simulink model "bh_SM_quad_NO_spin_props"  (R2017a)
settings: Solver=ode23t  StartTime=0.0  StopTime=200  FixedStep=0.001  RelTol=1e-5  EnableMultiTasking=on
undefined symbols (not defined in the file): P_elec, P_mot, P_one_prop, P_rot, P_veh, P_veh_no_props, sigbuilder_block, X, xme_dot_0, Y, Z
libraries: bh_6dof_LIBRARY x22, sm_lib x22, nesl_utility x19, simulink_extras x17, simulink x15
(part 3 of 3)

== system bh_SM_quad_NO_spin_props/CONT_SYS W_MOT_CMDS/MOTOR_sys/MOTOR_1/prefilter ==
  note: Y = U *     wn^2/( s^2 + 2*p*wn*s + wn^2)
      | Y*( s^2 + 2*p*wn*s + wn^2) = U * wn^2
      |
      | y'' + y'*2*p*wn + y*wn^2 = U*wn^2
  U : Inport
  Gain : Gain  Gain=2*p*wn
  Gain1 : Gain  Gain=wn^2
  Gain2 : Gain  Gain=wn^2
  Integrator : Integrator
  Integrator1 : Integrator
  Sum : Sum  Inputs=|+--
  U_filt : Outport
  U_DOT : Outport  Port=2
  wires:
  Integrator/1 -> Integrator1/1, [Y_DOT], Gain/1  "y_dot"
  Sum/1 -> Integrator/1  "y_dot_dot"
  Integrator1/1 -> Gain1/1, U_filt/1  "y"
  U/1 -> Gain2/1
  Gain2/1 -> Sum/1
  Gain/1 -> Sum/3
  Gain1/1 -> Sum/2
  [Y_DOT] -> U_DOT/1

== system bh_SM_quad_NO_spin_props/CONT_SYS W_MOT_CMDS/MOTOR_sys/MOTOR_2/prefilter ==
  note: Y = U *     wn^2/( s^2 + 2*p*wn*s + wn^2)
      | Y*( s^2 + 2*p*wn*s + wn^2) = U * wn^2
      |
      | y'' + y'*2*p*wn + y*wn^2 = U*wn^2
  U : Inport
  Gain : Gain  Gain=2*p*wn
  Gain1 : Gain  Gain=wn^2
  Gain2 : Gain  Gain=wn^2
  Integrator : Integrator
  Integrator1 : Integrator
  Sum : Sum  Inputs=|+--
  U_filt : Outport
  U_DOT : Outport  Port=2
  wires:
  Integrator/1 -> Integrator1/1, [Y_DOT], Gain/1  "y_dot"
  Sum/1 -> Integrator/1  "y_dot_dot"
  Integrator1/1 -> Gain1/1, U_filt/1  "y"
  U/1 -> Gain2/1
  Gain2/1 -> Sum/1
  Gain/1 -> Sum/3
  Gain1/1 -> Sum/2
  [Y_DOT] -> U_DOT/1

== system bh_SM_quad_NO_spin_props/CONT_SYS W_MOT_CMDS/MOTOR_sys/MOTOR_3/prefilter ==
  note: Y = U *     wn^2/( s^2 + 2*p*wn*s + wn^2)
      | Y*( s^2 + 2*p*wn*s + wn^2) = U * wn^2
      |
      | y'' + y'*2*p*wn + y*wn^2 = U*wn^2
  U : Inport
  Gain : Gain  Gain=2*p*wn
  Gain1 : Gain  Gain=wn^2
  Gain2 : Gain  Gain=wn^2
  Integrator : Integrator
  Integrator1 : Integrator
  Sum : Sum  Inputs=|+--
  U_filt : Outport
  U_DOT : Outport  Port=2
  wires:
  Integrator/1 -> Integrator1/1, [Y_DOT], Gain/1  "y_dot"
  Sum/1 -> Integrator/1  "y_dot_dot"
  Integrator1/1 -> Gain1/1, U_filt/1  "y"
  U/1 -> Gain2/1
  Gain2/1 -> Sum/1
  Gain/1 -> Sum/3
  Gain1/1 -> Sum/2
  [Y_DOT] -> U_DOT/1

== system bh_SM_quad_NO_spin_props/CONT_SYS W_MOT_CMDS/MOTOR_sys/MOTOR_4/prefilter ==
  note: Y = U *     wn^2/( s^2 + 2*p*wn*s + wn^2)
      | Y*( s^2 + 2*p*wn*s + wn^2) = U * wn^2
      |
      | y'' + y'*2*p*wn + y*wn^2 = U*wn^2
  U : Inport
  Gain : Gain  Gain=2*p*wn
  Gain1 : Gain  Gain=wn^2
  Gain2 : Gain  Gain=wn^2
  Integrator : Integrator
  Integrator1 : Integrator
  Sum : Sum  Inputs=|+--
  U_filt : Outport
  U_DOT : Outport  Port=2
  wires:
  Integrator/1 -> Integrator1/1, [Y_DOT], Gain/1  "y_dot"
  Sum/1 -> Integrator/1  "y_dot_dot"
  Integrator1/1 -> Gain1/1, U_filt/1  "y"
  U/1 -> Gain2/1
  Gain2/1 -> Sum/1
  Gain/1 -> Sum/3
  Gain1/1 -> Sum/2
  [Y_DOT] -> U_DOT/1

== system bh_SM_quad_NO_spin_props/MODEL_SYS/bh_6DOF (Simscape)/6DOF_JOINT_SYS/Angular_MEAS ==
  note: NOTE:  For the Transform sensor  block
      | Tthe DCM is:   r_BASE = R * r_FOLLOWER
  note: NOTE:  For the Transform sensor  block
      | The angular velocities are resolved into FOLLOWER frame components
  Calc Euler_rates : Subsystem
  Gain : Gain
  Math Function : Math  Operator=transpose  SaturateOnIntegerOverflow=on
  Mux : Mux  Inputs=3
  PS-Simulink Converter1 : nesl_utility/PS-Simulink Converter  PhysicalDomain=network_engine_domain  SubClassName=ps_output  LeftPortType=input  RightPortType=output  PseudoPeriodic=off  Frequencies=[]  Unit=rad/s  AffineConversion=off
  PS-Simulink Converter2 : nesl_utility/PS-Simulink Converter  PhysicalDomain=network_engine_domain  SubClassName=ps_output  LeftPortType=input  RightPortType=output  PseudoPeriodic=off  Frequencies=[]  Unit=rad/s  AffineConversion=off
  PS-Simulink Converter6 : nesl_utility/PS-Simulink Converter  PhysicalDomain=network_engine_domain  SubClassName=ps_output  LeftPortType=input  RightPortType=output  PseudoPeriodic=off  Frequencies=[]  Unit=1  AffineConversion=off
  PS-Simulink Converter7 : nesl_utility/PS-Simulink Converter  PhysicalDomain=network_engine_domain  SubClassName=ps_output  LeftPortType=input  RightPortType=output  PseudoPeriodic=off  Frequencies=[]  Unit=rad/s  AffineConversion=off
  Reshape1 : Reshape  OutputDimensionality=Column vector (2-D)
  Reshape2 : Reshape  OutputDimensionality=Column vector (2-D)
  Reshape3 : Reshape  OutputDimensionality=Column vector (2-D)
  Transform Sensor : sm_lib/Frames and Transforms/Transform Sensor  MeasurementFrame=Base  SenseAngle=off  SenseAxis=off  SenseAngle1=off  SenseAngle2=off  SenseAngle3=off  SenseQ=off  SenseR=on  SenseOmegaX=off  SenseOmegaY=off  SenseOmegaZ=off  SenseOmega1=off  SenseOmega2=off  SenseOmega3=off  SenseQDot=off  SenseRDot=off  SenseAlphaX=off  SenseAlphaY=off  SenseAlphaZ=off  SenseAlpha1=off  SenseAlpha2=off  SenseAlpha3=off  SenseQDDot=off  SenseRDDot=off  SenseX=off  SenseY=off  SenseZ=off  SenseRad=off  SenseAzim=off  SenseDist=off  SenseInc=off  SenseXDot=off  SenseYDot=off  SenseZDot=off  SenseRadDot=off  SenseAzimDot=off  SenseDistDot=off  SenseIncDot=off  SenseXDDot=off  SenseYDDot=off  SenseZDDot=off  SenseRadDDot=off  SenseAzimDDot=off  SenseDistDDot=off  SenseIncDDot=off
  Transform Sensor1 : sm_lib/Frames and Transforms/Transform Sensor  MeasurementFrame=Follower  SenseAngle=off  SenseAxis=off  SenseAngle1=off  SenseAngle2=off  SenseAngle3=off  SenseQ=off  SenseR=off  SenseOmegaX=on  SenseOmegaY=on  SenseOmegaZ=on  SenseOmega1=off  SenseOmega2=off  SenseOmega3=off  SenseQDot=off  SenseRDot=off  SenseAlphaX=off  SenseAlphaY=off  SenseAlphaZ=off  SenseAlpha1=off  SenseAlpha2=off  SenseAlpha3=off  SenseQDDot=off  SenseRDDot=off  SenseX=off  SenseY=off  SenseZ=off  SenseRad=off  SenseAzim=off  SenseDist=off  SenseInc=off  SenseXDot=off  SenseYDot=off  SenseZDot=off  SenseRadDot=off  SenseAzimDot=off  SenseDistDot=off  SenseIncDot=off  SenseXDDot=off  SenseYDDot=off  SenseZDDot=off  SenseRadDDot=off  SenseAzimDDot=off  SenseDistDDot=off  SenseIncDDot=off
  calc_DCM : MATLAB Function  TreatAsAtomicUnit=on
  B : PMIOPort  Port=1  Side=Left
  F : PMIOPort  Port=2  Side=Right
  wb : Outport
  bRg : Outport  Port=2
  eul : Outport  Port=3
  eul_rates : Outport  Port=4
  wires:
  PS-Simulink Converter6/1 -> Gain/1  "BRF"
  PS-Simulink Converter7/1 -> Mux/1
  PS-Simulink Converter1/1 -> Mux/2
  PS-Simulink Converter2/1 -> Mux/3
  Gain/1 -> Math Function/1  "gRb"
  Math Function/1 -> [bRg], bRg/1  "bRg"
  Mux/1 -> Reshape1/1
  [bRg] -> calc_DCM/1(bRg)
  calc_DCM/1(eul_vec) -> Reshape2/1
  Reshape2/1 -> [e], eul/1
  Calc Euler_rates/1(Euler_rates) -> Reshape3/1
  Reshape3/1 -> eul_rates/1
  Reshape1/1 -> [wb], wb/1
  [wb] -> Calc Euler_rates/1("p q r ")
  [e] -> Calc Euler_rates/2(Euler_angs)
  connections:
  PS-Simulink Converter7/LConn1 -- Transform Sensor1/RConn2
  PS-Simulink Converter6/LConn1 -- Transform Sensor/RConn2
  Transform Sensor1/RConn1 -- Transform Sensor/RConn1 -- F/RConn1
  Transform Sensor/LConn1 -- B/RConn1 -- Transform Sensor1/LConn1
  PS-Simulink Converter2/LConn1 -- Transform Sensor1/RConn4
  Transform Sensor1/RConn3 -- PS-Simulink Converter1/LConn1

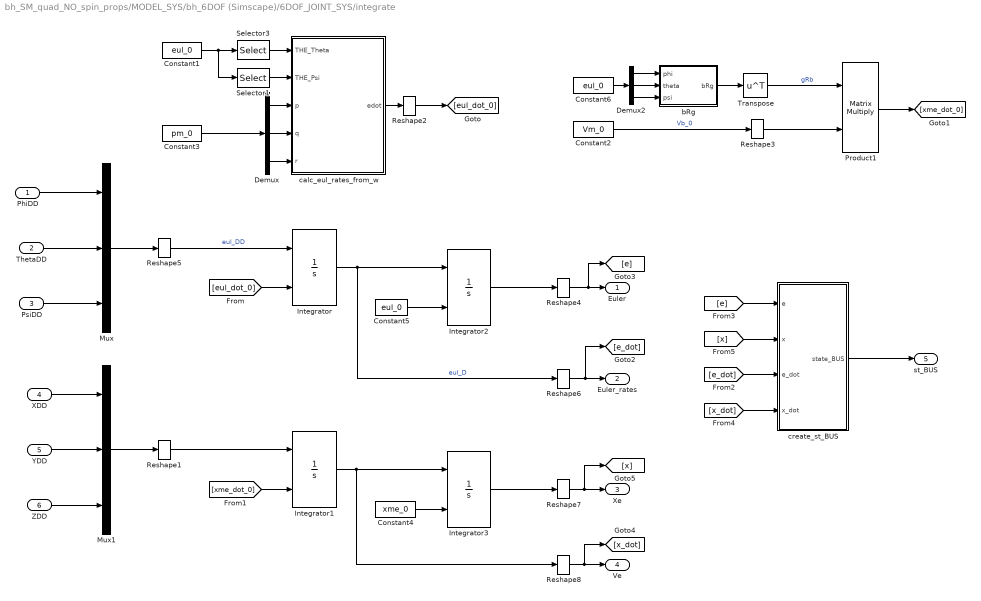
== system bh_SM_quad_NO_spin_props/MODEL_SYS/bh_6DOF (Simscape)/6DOF_JOINT_SYS/integrate ==
  PhiDD : Inport
  ThetaDD : Inport  Port=2
  PsiDD : Inport  Port=3
  XDD : Inport  Port=4
  YDD : Inport  Port=5
  ZDD : Inport  Port=6
  Constant1 : Constant  Value=eul_0  OutDataTypeStr=Inherit: Inherit via back propagation
  Constant2 : Constant  Value=Vm_0  OutDataTypeStr=Inherit: Inherit via back propagation
  Constant3 : Constant  Value=pm_0  OutDataTypeStr=Inherit: Inherit via back propagation
  Constant4 : Constant  Value=xme_0  OutDataTypeStr=Inherit: Inherit via back propagation
  Constant5 : Constant  Value=eul_0  OutDataTypeStr=Inherit: Inherit via back propagation
  Constant6 : Constant  Value=eul_0  OutDataTypeStr=Inherit: Inherit via back propagation
  Demux : Demux  Outputs=3
  Demux2 : Demux  Outputs=3
  Integrator : Integrator  InitialConditionSource=external  ContinuousStateAttributes={'DOT_phi', 'DOT_theta','DOT_psi'}
      settings: AttributesFormatString=%<ContinuousStateAttributes>
  Integrator1 : Integrator  InitialConditionSource=external  ContinuousStateAttributes={'DOT_Xe', 'DOT_Ye', 'DOT_Ze'}
      settings: AttributesFormatString=%<ContinuousStateAttributes>
  Integrator2 : Integrator  InitialConditionSource=external  ContinuousStateAttributes={'phi', 'theta','psi'}
      settings: AttributesFormatString=%<ContinuousStateAttributes>
  Integrator3 : Integrator  InitialConditionSource=external  ContinuousStateAttributes={'Xe', 'Ye', 'Ze'}
      settings: AttributesFormatString=%<ContinuousStateAttributes>
  Mux : Mux  Inputs=3
  Mux1 : Mux  Inputs=3
  Product1 : Product  Multiplication=Matrix(*)  SaturateOnIntegerOverflow=on  InputSameDT=on  OutDataTypeStr=Inherit: Same as first input
  Reshape{1..8} (8 alike) : Reshape  OutputDimensionality=Column vector (2-D)
  Selector1 : Selector  InputPortWidth=3  IndexOptions=Index vector (dialog)  Indices=3  OutputSizes=1
  Selector3 : Selector  InputPortWidth=3  IndexOptions=Index vector (dialog)  Indices=2  OutputSizes=1
  Transpose : Math  Operator=transpose  SaturateOnIntegerOverflow=on
  bRg : MATLAB Function  TreatAsAtomicUnit=on
  calc_eul_rates_from_w : MATLAB Function  TreatAsAtomicUnit=on
  create_st_BUS : Subsystem
  Euler : Outport
  Euler_rates : Outport  Port=2
  Xe : Outport  Port=3
  Ve : Outport  Port=4
  st_BUS : Outport  Port=5
  wires:
  PhiDD/1 -> Mux/1
  ThetaDD/1 -> Mux/2
  PsiDD/1 -> Mux/3
  Mux/1 -> Reshape5/1
  XDD/1 -> Mux1/1
  YDD/1 -> Mux1/2
  ZDD/1 -> Mux1/3
  Mux1/1 -> Reshape1/1
  Integrator1/1 -> Reshape8/1, Integrator3/1
  Integrator/1 -> Reshape6/1, Integrator2/1  "eul_D"
  Reshape5/1 -> Integrator/1  "eul_DD"
  Reshape1/1 -> Integrator1/1
  Constant5/1 -> Integrator2/2
  Constant1/1 -> Selector1/1, Selector3/1
  [eul_dot_0] -> Integrator/2
  Constant4/1 -> Integrator3/2
  Constant2/1 -> Reshape3/1  "Vb_0"
  bRg/1(bRg) -> Transpose/1
  Reshape3/1 -> Product1/2
  Constant6/1 -> Demux2/1
  Transpose/1 -> Product1/1  "gRb"
  Product1/1 -> [xme_dot_0]
  [xme_dot_0] -> Integrator1/2
  Integrator3/1 -> Reshape7/1
  Integrator2/1 -> Reshape4/1
  Reshape4/1 -> [e], Euler/1
  Reshape6/1 -> [e_dot], Euler_rates/1
  Reshape7/1 -> [x], Xe/1
  Reshape8/1 -> [x_dot], Ve/1
  Demux2/1 -> bRg/1(phi)
  Demux2/2 -> bRg/2(theta)
  Demux2/3 -> bRg/3(psi)
  Selector3/1 -> calc_eul_rates_from_w/1(THE_Theta)
  Selector1/1 -> calc_eul_rates_from_w/2(THE_Psi)
  Demux/3 -> calc_eul_rates_from_w/5(r)
  Demux/2 -> calc_eul_rates_from_w/4(q)
  Demux/1 -> calc_eul_rates_from_w/3(p)
  calc_eul_rates_from_w/1(edot) -> Reshape2/1
  Constant3/1 -> Demux/1
  Reshape2/1 -> [eul_dot_0]
  [e] -> create_st_BUS/1(e)
  [x] -> create_st_BUS/2(x)
  [e_dot] -> create_st_BUS/3(e_dot)
  [x_dot] -> create_st_BUS/4(x_dot)
  create_st_BUS/1(state_BUS) -> st_BUS/1

== system bh_SM_quad_NO_spin_props/MODEL_SYS/bh_6DOF (Simscape)/6DOF_JOINT_SYS/Angular_MEAS/Calc Euler_rates ==
  "p q r " : Inport
  Euler_angs : Inport  Port=2
  Demux1 : Demux  Outputs=3
  Demux2 : Demux  Outputs=3
  Demux3 : Demux  Outputs=3
  Mux1 : Mux  Inputs=3
  Reshape1 : Reshape  OutputDimensionality=Column vector (2-D)
  Reshape2 : Reshape  OutputDimensionality=Column vector (2-D)
  Terminator : Terminator
  my_euler_rates : MATLAB Function  TreatAsAtomicUnit=on
  Euler_rates : Outport
  wires:
  Reshape1/1 -> Demux3/1  "wb"
  my_euler_rates/1(euler_rates) -> Demux2/1  "euler_rates"
  Demux2/3 -> Mux1/3  "psidot_X3_roll"
  Demux2/2 -> Mux1/2  "thetadot_Y2_pitch"
  Demux2/1 -> Mux1/1  "phidot_Z1_yaw"
  Reshape2/1 -> Euler_rates/1
  Mux1/1 -> Reshape2/1
  Demux3/3 -> my_euler_rates/5(r)
  Demux3/2 -> my_euler_rates/4(q)
  Demux3/1 -> my_euler_rates/3(p)
  Euler_angs/1 -> Demux1/1
  "p q r "/1 -> Reshape1/1
  Demux1/2 -> my_euler_rates/1(theta)  "theta"
  Demux1/1 -> Terminator/1  "phi"
  Demux1/3 -> my_euler_rates/2(psi)  "psi"

== system bh_SM_quad_NO_spin_props/MODEL_SYS/bh_6DOF (Simscape)/6DOF_JOINT_SYS/integrate/create_st_BUS ==
  e : Inport
  x : Inport  Port=2
  e_dot : Inport  Port=3
  x_dot : Inport  Port=4
  Bus Creator : BusCreator  Inputs=4
  Bus Creator1 : BusCreator  Inputs=6
  Bus Creator2 : BusCreator  Inputs=6
  Demux{,1..3} (4 alike) : Demux  Outputs=3
  Mux : Mux  Inputs=2
  Mux1 : Mux  Inputs=2
  Reshape1 : Reshape  OutputDimensionality=Column vector (2-D)
  Reshape8 : Reshape  OutputDimensionality=Column vector (2-D)
  state_BUS : Outport
  wires:
  e/1 -> Mux/1, [e]
  x/1 -> Mux/2, [x]
  e_dot/1 -> Mux1/1, [eD]
  x_dot/1 -> Mux1/2, [xD]
  Mux1/1 -> Reshape1/1
  Mux/1 -> Reshape8/1
  Reshape1/1 -> Bus Creator/2  "vel_col"
  Reshape8/1 -> Bus Creator/1  "pos_col"
  Bus Creator1/1 -> Bus Creator/3  "Pos_list"
  Demux/1 -> Bus Creator1/1  "Phi"
  Demux/2 -> Bus Creator1/2  "Theta"
  Demux/3 -> Bus Creator1/3  "Psi"
  Demux1/2 -> Bus Creator1/5  "Y"
  Demux1/3 -> Bus Creator1/6  "Z"
  Demux1/1 -> Bus Creator1/4  "X"
  [e] -> Demux/1
  [x] -> Demux1/1
  Bus Creator2/1 -> Bus Creator/4  "Vel_list"
  Demux2/1 -> Bus Creator2/1  "Phi_D"
  Demux2/2 -> Bus Creator2/2  "Theta_D"
  Demux2/3 -> Bus Creator2/3  "Psi_D"
  Demux3/1 -> Bus Creator2/4  "X_D"
  Demux3/2 -> Bus Creator2/5  "Y_D"
  Demux3/3 -> Bus Creator2/6  "Z_D"
  [eD] -> Demux2/1
  [xD] -> Demux3/1
  Bus Creator/1 -> state_BUS/1

== matlab function bh_SM_quad_NO_spin_props/MODEL_SYS/bh_6DOF (Simscape)/6DOF_JOINT_SYS/integrate/bRg ==
  data: phi input; bRg output; theta input; psi input
function bRg = bRg(phi,theta,psi)
%#codegen

%    This function was generated by the Symbolic Math Toolbox version 7.2.
%    28-Aug-2017 10:05:16

bRg = reshape([cos(phi).*cos(theta),-cos(psi).*sin(phi)+cos(phi).*sin(psi).*sin(theta),sin(phi).*sin(psi)+cos(phi).*cos(psi).*sin(theta),cos(theta).*sin(phi),cos(phi).*cos(psi)+sin(phi).*sin(psi).*sin(theta),-cos(phi).*sin(psi)+cos(psi).*sin(phi).*sin(theta),-sin(theta),cos(theta).*sin(psi),cos(psi).*cos(theta)],[3,3]);

== matlab function bh_SM_quad_NO_spin_props/CONT_SYS W_MOT_CMDS/FM_to_w2 ==
  data: L input; w2_cmd output; Thrust_const input; Twist_const input; Thrust input; TQ_roll_X input; TQ_pit_Y input; TQ_yaw_Z input
function w2_cmd = FMtow2(L, Thrust_const, Twist_const, Thrust, TQ_roll_X, TQ_pit_Y, TQ_yaw_Z)
%#codegen

    % simplify the variable names
    b = Thrust_const;
    k = Twist_const;

    % construct the co-efficient matrix:
    %  F_and_M = C * w^2
    %
    % C = [     b,    b,    b,    b;
    %           0,    b*L,  0,   -b*L;
    %          -b*L,  0,    b*L,  0;
    %          -k,    k,   -k,    k; ];

    % used Symbolic toolbox to compute inv(C)
    C_inv = [
             1/(4*b),          0, -1/(2*L*b), -1/(4*k);
             1/(4*b),  1/(2*L*b),          0,  1/(4*k);
             1/(4*b),          0,  1/(2*L*b), -1/(4*k);
             1/(4*b), -1/(2*L*b),          0,  1/(4*k);
            ];
    % solve for the w^2 vec
    F_and_M_col = [Thrust, TQ_roll_X, TQ_pit_Y, TQ_yaw_Z].' ;

    w2_cmd = C_inv * F_and_M_col;
    
    tf_col = (w2_cmd >= 0);
   assert(all(w2_cmd), 'ERROR: some w2 are NEGATIVE !')
   %assert(false, 'ERROR: some w2 are NEGATIVE !')
end

== matlab function bh_SM_quad_NO_spin_props/a_circle1/MATLAB Function ==
  data: t_clock input; XYZ output; t_to_start input; RADIUS input; ztgt input; w input
function XYZ = fcn(t_clock, t_to_start, RADIUS, ztgt, w)

t    = t_clock - t_to_start;

theta = w*t;

x = RADIUS * cos(theta);
y = RADIUS * sin(theta);
z = ztgt;


XYZ = [x;y;z];

== matlab function bh_SM_quad_NO_spin_props/CONT_SYS Force_Moment_CMDS/PITCH_and_ROLL_CONT/MATLAB Function ==
  data: Gr input size=[2 1]; Qr output size=[2 1]; ang input size=[1 1]
function Qr = fcn(Gr, ang)
%#codegen

    bRg = [  cos(ang),  sin(ang);
            -sin(ang),  cos(ang);
          ];  

    Qr = bRg * Gr;
end

== matlab function bh_SM_quad_NO_spin_props/MODEL_SYS/bh_6DOF (Simscape)/6DOF_JOINT_SYS/Angular_MEAS/Calc Euler_rates/my_euler_rates ==
  data: theta input; euler_rates output; psi input; p input; q input; r input
function euler_rates = my_euler_rates(theta,psi,p,q,r)
%#codegen

%    This function was generated by the Symbolic Math Toolbox version 7.0.
%    09-Jun-2016 10:28:25

euler_rates = [(r.*cos(psi)+q.*sin(psi))./cos(theta);
                q.*cos(psi)-r.*sin(psi);
               (p.*cos(theta)+r.*cos(psi).*sin(theta)+q.*sin(psi).*sin(theta))./cos(theta)];

== matlab function bh_SM_quad_NO_spin_props/MODEL_SYS/bh_6DOF (Simscape)/6DOF_JOINT_SYS/integrate/calc_eul_rates_from_w ==
  data: THE_Theta input; edot output; THE_Psi input; p input; q input; r input
function edot = calc_eul_rates_from_w(THE_Theta,THE_Psi,p,q,r)
%#codegen

%    This function was generated by the Symbolic Math Toolbox version 7.2.
%    28-Aug-2017 10:05:22

edot = [(r.*cos(THE_Psi)+q.*sin(THE_Psi))./cos(THE_Theta);q.*cos(THE_Psi)-r.*sin(THE_Psi);(p.*cos(THE_Theta)+r.*cos(THE_Psi).*sin(THE_Theta)+q.*sin(THE_Psi).*sin(THE_Theta))./cos(THE_Theta)];

== matlab function bh_SM_quad_NO_spin_props/MODEL_SYS/bh_6DOF (Simscape)/6DOF_JOINT_SYS/Angular_MEAS/calc_DCM ==
  data: bRg input; eul_vec output
function eul_vec = calc_eul_ang(bRg)
%#codegen

% bRg = [ ...
%                               cos(phi)*cos(theta),                              cos(theta)*sin(phi),         -sin(theta);
%  cos(phi)*sin(psi)*sin(theta) - cos(psi)*sin(phi), cos(phi)*cos(psi) + sin(phi)*sin(psi)*sin(theta), cos(theta)*sin(psi);
%  sin(phi)*sin(psi) + cos(phi)*cos(psi)*sin(theta), cos(psi)*sin(phi)*sin(theta) - cos(phi)*sin(psi), cos(psi)*cos(theta);
%  ];

%phi, theta, psi


theta = asin( -bRg(1,3)  ); %  theta is in the range [-pi/2, pi/2]

% Recall the DOC on atan2()
%     atan2(Y,X) is the four quadrant arctangent of the elements of X and Y
%     such that -pi <= atan2(Y,X) <= pi

Y   = bRg(1,2);
X   = bRg(1,1);
phi = atan2(Y,X);

Y   = bRg(2,3);
X   = bRg(3,3);
psi = atan2(Y,X);

% now populate the output
eul_vec    = zeros(3,1);

eul_vec(1) = phi;
eul_vec(2) = theta;
eul_vec(3) = psi;

end

== matlab function bh_SM_quad_NO_spin_props/CONT_SYS W_MOT_CMDS/w2toFM1 ==
  data: L input; Tbz_col output; Thrust_const input; Twist_const input; w2_col input; Mbz_col output; wM_col output
function [Tbz_col, Mbz_col, wM_col] = w2toFM(L, Thrust_const, Twist_const, w2_col)
%#codegen

    % simplify the variable names
    b = Thrust_const;
    k = Twist_const;

    % construct the co-efficient matrix:
    %  F_and_M = C * w^2
    
%     C = [     b,    b,    b,    b;
%               0,    b*L,  0,   -b*L;
%              -b*L,  0,    b*L,  0;
%              -k,    k,   -k,    k; ];

    Tbz_col = [ b; b; b; b ]  .*  w2_col;     
    Mbz_col = [-k; k;-k; k ]  .*  w2_col;          
    wM_col  = [ 1;-1; 1;-1 ]  .*  sqrt(w2_col); 
end

== matlab function bh_SM_quad_NO_spin_props/CONT_SYS W_MOT_CMDS/w2toFM2 ==
  data: L input; Thrust output; Thrust_const input; Twist_const input; w2_col input; TQ_roll_X output; TQ_pit_Y output; TQ_yaw_Z output
function [Thrust, TQ_roll_X, TQ_pit_Y, TQ_yaw_Z] = w2toFM(L, Thrust_const, Twist_const, w2_col)
%#codegen

    % simplify the variable names
    b = Thrust_const;
    k = Twist_const;

    % construct the co-efficient matrix:
    %  F_and_M = C * w^2
    
    C = [     b,    b,    b,    b;
              0,    b*L,  0,   -b*L;
             -b*L,  0,    b*L,  0;
             -k,    k,   -k,    k; ];

    % solve for the FM_col
    %   FM_col = [Thrust, TQ_roll_X, TQ_pit_Y, TQ_yaw_Z].' ;
    
    FM_col  =  C * w2_col;
    
    Thrust    =  FM_col(1);
    TQ_roll_X =  FM_col(2);
    TQ_pit_Y  =  FM_col(3);
    TQ_yaw_Z  =  FM_col(4);
    
end
